simulink model "ten"  (R2025b)
settings: Solver=VariableStepAuto  StartTime=0.0  StopTime=20  RelTol=1e-3
settings Model: Creator=allen  LastModifiedBy=allen

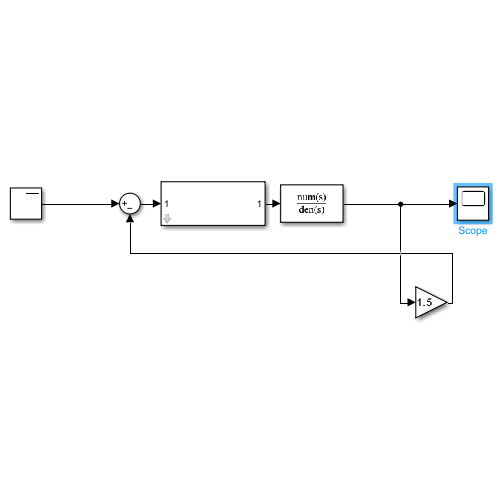
[thumbnail: Simulink's stored preview of the top-level diagram]
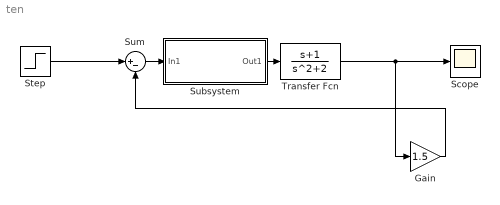
== system ten ==
  Gain : Gain  Gain=1.5
  Scope : Scope
      settings: ActiveDisplayYMinimum=-0.56814128187738855  ActiveDisplayYMaximum=1.250908075689342
  Step : Step  SampleTime=0
  Subsystem : Subsystem  mask{Kp=1, Ki=1, Kd=0.1}
      mask prompts: Kp "比例系数"; Ki "积分系数"; Kd "微分系数"
      mask DialogControl ParameterGroupVar Prompt: 参数
  Sum : Sum  Inputs=|+-
  Transfer Fcn : TransferFcn  Numerator=[1 1]  Denominator=[1 0 2]
  wires:
  Step/1 -> Sum/1
  Gain/1 -> Sum/2
  Transfer Fcn/1 -> Gain/1, Scope/1
  Sum/1 -> Subsystem/1(In1)
  Subsystem/1(Out1) -> Transfer Fcn/1

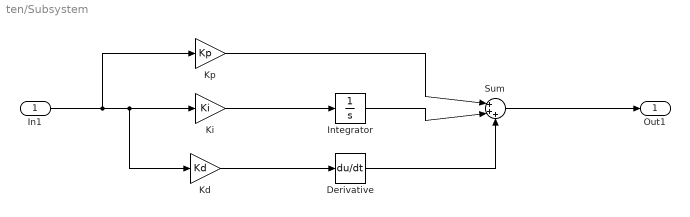
== system ten/Subsystem ==
  In1 : Inport
  Derivative : Derivative
  Integrator : Integrator
  Kd : Gain  Gain=Kd
  Ki : Gain  Gain=Ki
  Kp : Gain  Gain=Kp
  Sum : Sum  Inputs=|+++
  Out1 : Outport
  wires:
  In1/1 -> Kp/1, Kd/1, Ki/1
  Ki/1 -> Integrator/1
  Kp/1 -> Sum/1
  Integrator/1 -> Sum/2
  Kd/1 -> Derivative/1
  Derivative/1 -> Sum/3
  Sum/1 -> Out1/1
